simulink model "thermal_system"  (R2024b)
settings: Solver=VariableStepAuto  StartTime=0.0  StopTime=20000  MaxStep=0.01  RelTol=1e-3
undefined symbols (not defined in the file): C, Q, T_a, T_setpoint, U
libraries: simulink x1
settings Model: Creator=Utilizador  LastModifiedBy=Utilizador
settings SolverCC: ZeroCrossAlgorithm=Adaptive
settings DebuggingCC: IgnoredZcDiagnostic=none

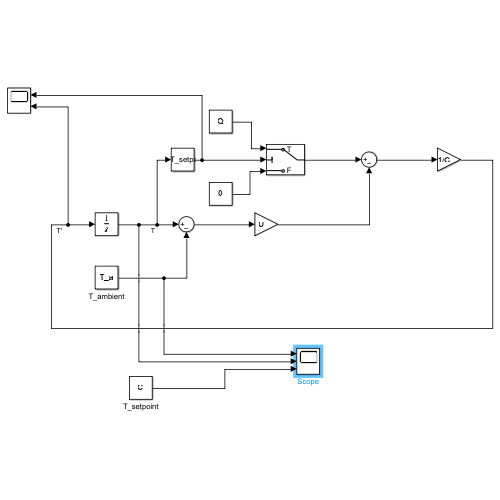
[thumbnail: Simulink's stored preview of the top-level diagram]
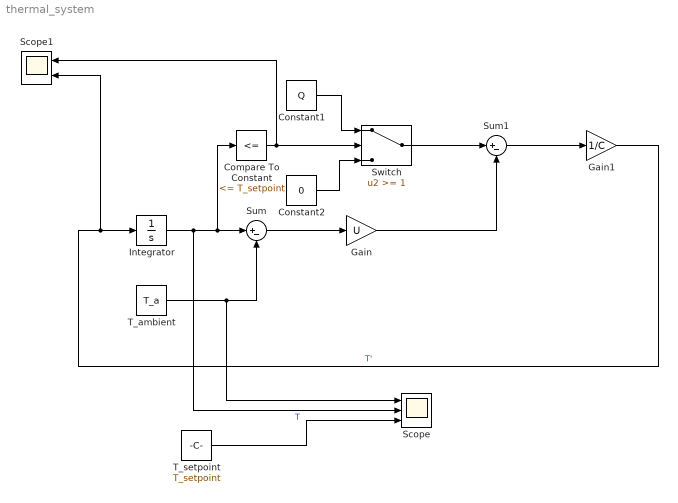
== system thermal_system ==
  Compare To Constant : simulink/Logic and Bit Operations/Compare To Constant  relop=<=  const=T_setpoint  OutDataTypeStr=boolean
  Constant1 : Constant  Value=Q
  Constant2 : Constant  Value=0
  Gain : Gain  Gain=U
  Gain1 : Gain  Gain=1/C
  Integrator : Integrator
  Scope : Scope  NumInputPorts=3
  Scope1 : Scope  NumInputPorts=2
  Sum : Sum  Inputs=|+-
  Sum1 : Sum  Inputs=|+-
  Switch : Switch  Threshold=1  SaturateOnIntegerOverflow=off  InputSameDT=off
  T_ambient : Constant  Value=T_a
  T_setpoint : Constant  Value=T_setpoint
  wires:
  Integrator/1 -> Scope/2, Compare To Constant/1, Sum/1  "T"
  Gain1/1 -> Scope1/2, Integrator/1  "T'"
  T_ambient/1 -> Scope/1, Sum/2
  Sum/1 -> Gain/1
  Gain/1 -> Sum1/2
  Sum1/1 -> Gain1/1
  Switch/1 -> Sum1/1
  Constant1/1 -> Switch/1
  Constant2/1 -> Switch/3
  Compare To Constant/1 -> Switch/2, Scope1/1
  T_setpoint/1 -> Scope/3
